simulink model "power_steppermotor_input_forschem"  (R2015b)
settings: Solver=FixedStepDiscrete  StartTime=0.0  StopTime=0.35  FixedStep=Ts  MaxStep=2e-6
PreLoadFcn:
  | assignin('base','Ts',1e-8);
InitFcn:
  | Ts=1e-8;
undefined symbols (not defined in the file): DiscIntNeverNeededParam
libraries: powerlib x1
Description:
  | Copyright 2008-2015 The MathWorks, Inc.
settings Model: ExtModeAutoUpdateStatusClock=off  Creator=MathWorks  LastModifiedBy=YogurtSuee
settings DataIOCC: SaveFormat=Array  SignalLoggingSaveFormat=ModelDataLogs
settings OptimizationCC: ExpressionDepthLimit=2147483647  InitFltsAndDblsToZero=on
settings DebuggingCC: UnderspecifiedInitializationDetection=Classic  MergeDetectMultiDrivingBlocksExec=none  SignalResolutionControl=TryResolveAllWithWarning  SolverPrmCheckMsg=warning  FcnCallInpInsideContextMsg=UseLocalSettings  StateNameClashWarn=warning
settings HardwareCC: ProdBitPerPointer=32  ProdLargestAtomicFloat=None  ProdIntDivRoundTo=Undefined  ProdEndianess=Unspecified  ProdWordSize=32  ProdHWDeviceType=32-bit Generic
settings GRTTargetCC: GeneratePreprocessorConditionals=Disable all  CombineOutputUpdateFcns=off  GRTInterface=on
settings ConfigComp: CovModelRefEnable=Off  CovSFcnEnable=off

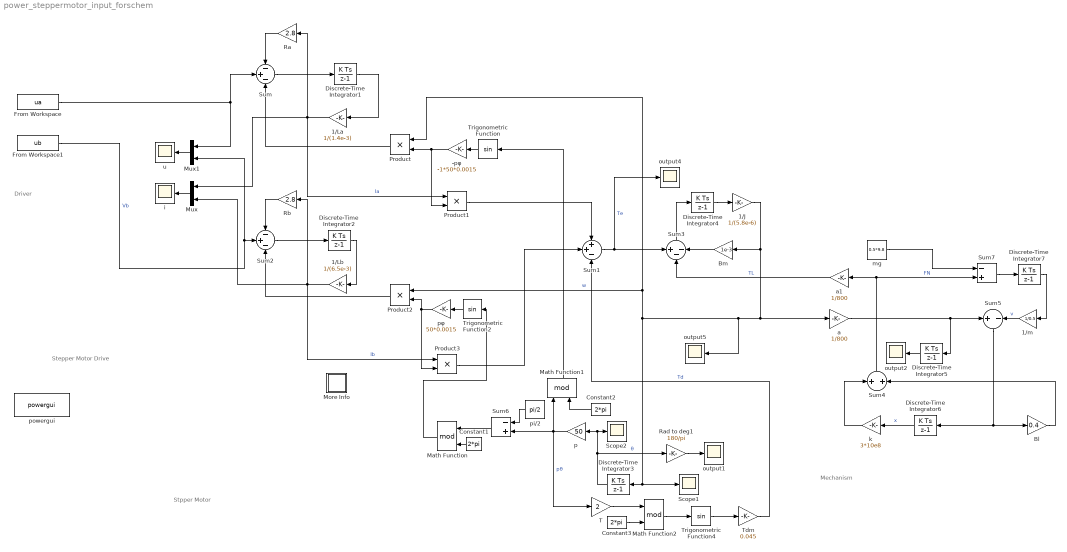
== system power_steppermotor_input_forschem ==
  note: Driver
  note: Stepper Motor Drive
  note: Stpper Motor
  note: Mechanism
  -pφ : Gain  Gain=-1*50*0.0015
  1/J : Gain  Gain=1/(5.8e-6)
  1/La : Gain  Gain=1/(1.4e-3)
  1/Lb : Gain  Gain=1/(6.5e-3)
  1/m : Gain  Gain=1/0.5
  Bl : Gain  Gain=0.4
  Bm : Gain  Gain=1e-3
  Constant1 : Constant  Value=2*pi
  Constant2 : Constant  Value=2*pi
  Constant3 : Constant  Value=2*pi
  Discrete-Time Integrator{1..7} (7 alike) : DiscreteIntegrator  SampleTime=Ts  ICPrevOutput=DiscIntNeverNeededParam  ICPrevScaledInput=DiscIntNeverNeededParam
  From Workspace : FromWorkspace  VariableName=ua  SampleTime=0
  From Workspace1 : FromWorkspace  VariableName=ub  SampleTime=0
  Math Function : Math  Operator=mod  SaturateOnIntegerOverflow=on
  Math Function1 : Math  Operator=mod  SaturateOnIntegerOverflow=on
  Math Function2 : Math  Operator=mod  SaturateOnIntegerOverflow=on
  More Info : Subsystem
      settings: OpenFcn=showdemo(bdroot(gcb))
      mask Display: disp('?')
  Mux : Mux  Inputs=2
  Mux1 : Mux  Inputs=2
  Product{,1..3} (4 alike) : Product
  Ra : Gain  Gain=2.8
  Rad to deg1 : Gain  Gain=180/pi
  Rb : Gain  Gain=2.8
  Scope1 : Scope
  Scope2 : Scope
  Sum : Sum  Inputs=-+-
  Sum1 : Sum  Inputs=++-
  Sum2 : Sum  Inputs=-+-
  Sum3 : Sum  Inputs=+--
  Sum4 : Sum
  Sum5 : Sum  Inputs=+-
  Sum6 : Sum  Inputs=-+
  Sum7 : Sum  Inputs=-+
  T : Gain  Gain=2
  Tdm : Gain  Gain=0.045
  Trigonometric Function : Trigonometry
  Trigonometric Function2 : Trigonometry
  Trigonometric Function4 : Trigonometry
  a : Gain  Gain=1/800
  a1 : Gain  Gain=1/800
  i : Scope
  k : Gain  Gain=3*10e8
  mg : Constant  Value=0.5*9.8
  output{1..2,4..5} (4 alike) : Scope
  p : Gain  Gain=50
  pi/2 : Constant  Value=pi/2
  powergui : powerlib/powergui  SimulationMode=Discrete  SolverType=Tustin/Backward Euler (TBE)  SampleTime=Ts  frequency=60  SPID=off  DisableSnubberDevices=off  DisableRonSwitches=off  DisableVfSwitches=off  SwTol=0  DisplayEquations=off  Interpol=off  ExternalGateDelay=off  methode=off  Ts=0  FunctionMessages=off  echomessages=off  HookPort=off  EnableUseOfTLC=off  x0status=blocks  frequencyindice=0  Pbase=100e6  ErrMax=1e-4  Iterations=50  UnitsV=V  UnitsW=W  buscounter=0  RestoreLinks=warning  ResistiveCurrentMeasurement=off  Frange=[0:2:500]  Ylog=off  Xlog=on  ShowGrid=off  save=off  variable=ZData  structure=0  ZoomFFT=on  StartTime=0.0  cycles=1  DisplayStyle=1  fundamental=60  FreqAxis=off  MaxFrequency=1000  frequencyindicesteady=1  RmsSteady=1  display=off
  pφ : Gain  Gain=50*0.0015
  u : Scope
  wires:
  Discrete-Time Integrator1/1 -> 1/La/1
  Sum/1 -> Discrete-Time Integrator1/1
  Ra/1 -> Sum/1
  1/La/1 -> Product1/1, Mux/1, Ra/1  "Ia"
  Product/1 -> Sum/3
  -pφ/1 -> Product/2, Product1/2
  Product1/1 -> Sum1/1
  Discrete-Time Integrator2/1 -> 1/Lb/1
  Sum2/1 -> Discrete-Time Integrator2/1
  Rb/1 -> Sum2/1
  1/Lb/1 -> Product3/1, Mux/2, Rb/1  "Ib"
  Product2/1 -> Sum2/3
  pφ/1 -> Product2/2, Product3/2
  Product3/1 -> Sum1/2
  Tdm/1 -> Sum1/3  "Td"
  1/J/1 -> output5/1, Product2/1, Product/1, Discrete-Time Integrator3/1, Scope1/1, a/1, Bm/1  "w"
  Sum3/1 -> Discrete-Time Integrator4/1
  Discrete-Time Integrator4/1 -> 1/J/1
  Discrete-Time Integrator3/1 -> Rad to deg1/1, Scope2/1, p/1  "θ"
  p/1 -> Sum6/2, T/1, Math Function1/1  "pθ"
  pi/2/1 -> Sum6/1
  Mux/1 -> i/1
  Mux1/1 -> u/1
  Trigonometric Function4/1 -> Tdm/1
  Constant1/1 -> Math Function/2
  Sum6/1 -> Math Function/1
  Math Function/1 -> Trigonometric Function2/1
  Constant2/1 -> Math Function1/2
  Math Function1/1 -> Trigonometric Function/1
  Constant3/1 -> Math Function2/2
  T/1 -> Math Function2/1
  Math Function2/1 -> Trigonometric Function4/1
  Sum1/1 -> output4/1, Sum3/1  "Te"
  Bm/1 -> Sum3/3
  Trigonometric Function/1 -> -pφ/1
  Trigonometric Function2/1 -> pφ/1
  From Workspace1/1 -> Mux1/2, Sum2/2  "Vb"
  From Workspace/1 -> Mux1/1, Sum/2
  Sum4/1 -> Sum7/2, a1/1  "FN"
  a/1 -> Discrete-Time Integrator5/1, Sum5/1
  mg/1 -> Sum7/1
  Sum7/1 -> Discrete-Time Integrator7/1
  Discrete-Time Integrator7/1 -> 1/m/1
  1/m/1 -> Sum5/2  "v"
  a1/1 -> Sum3/2  "TL"
  Sum5/1 -> Discrete-Time Integrator6/1, Bl/1
  Discrete-Time Integrator6/1 -> k/1  "x"
  k/1 -> Sum4/1
  Bl/1 -> Sum4/2
  Rad to deg1/1 -> output1/1
  Discrete-Time Integrator5/1 -> output2/1

== system power_steppermotor_input_forschem/More Info ==
